simulink model "NewKitchen_REB_workstation"  (R2020b)
settings: Solver=FixedStepAuto  StartTime=sim_start  StopTime=sim_end  FixedStep=sim_interval  RelTol=1e-3
undefined symbols (not defined in the file): AmbientTem, Power1, Power2, Power3, Velocity1, Velocity2
libraries: dspswit3 x6
(part 1 of 3)
settings Model: Creator=u2159176  LastModifiedBy=u2159176
settings DebuggingCC: UnconnectedInputMsg=none  UnconnectedOutputMsg=none  UnconnectedLineMsg=none  SFMachineParentedDataDiag=error
settings ModelReferenceCC: EnableRefExpFcnMdlSchedulingChecks=off

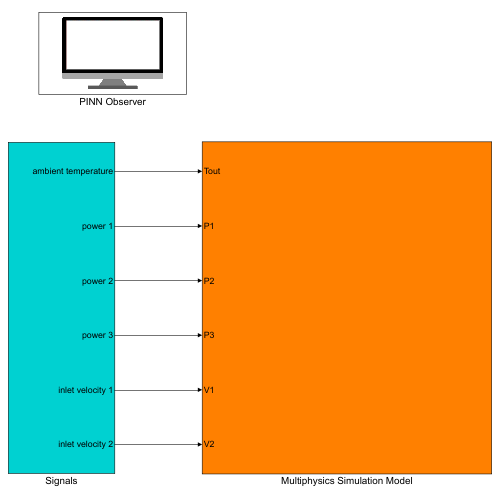
[thumbnail: Simulink's stored preview of the top-level diagram]
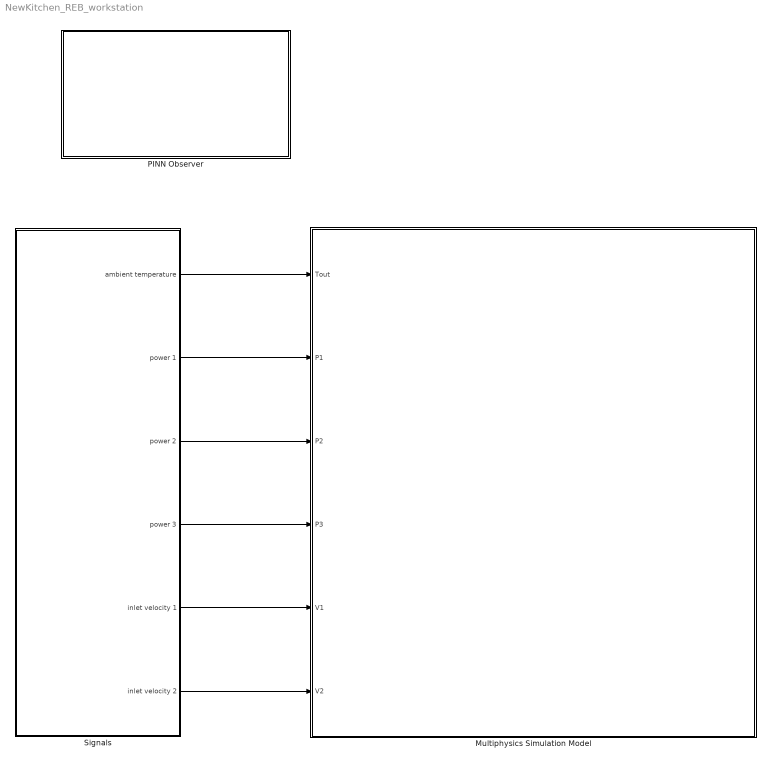
== system NewKitchen_REB_workstation ==
  Multiphysics Simulation Model : Subsystem
  PINN Observer : Subsystem
      mask Display: image('\\brio.ads.warwick.ac.uk\User68\u\u2159176\Desktop\comsol data\ECOS2023\tanshen\lcd_display.png'); % Use "Edit Image" on toolstrip to change.
  Signals : Subsystem
  wires:
  Signals/1(ambient temperature) -> Multiphysics Simulation Model/1(Tout)
  Signals/2(power 1) -> Multiphysics Simulation Model/2(P1)
  Signals/3(power 2) -> Multiphysics Simulation Model/3(P2)
  Signals/4(power 3) -> Multiphysics Simulation Model/4(P3)
  Signals/5(inlet velocity 1) -> Multiphysics Simulation Model/5(V1)
  Signals/6(inlet velocity 2) -> Multiphysics Simulation Model/6(V2)

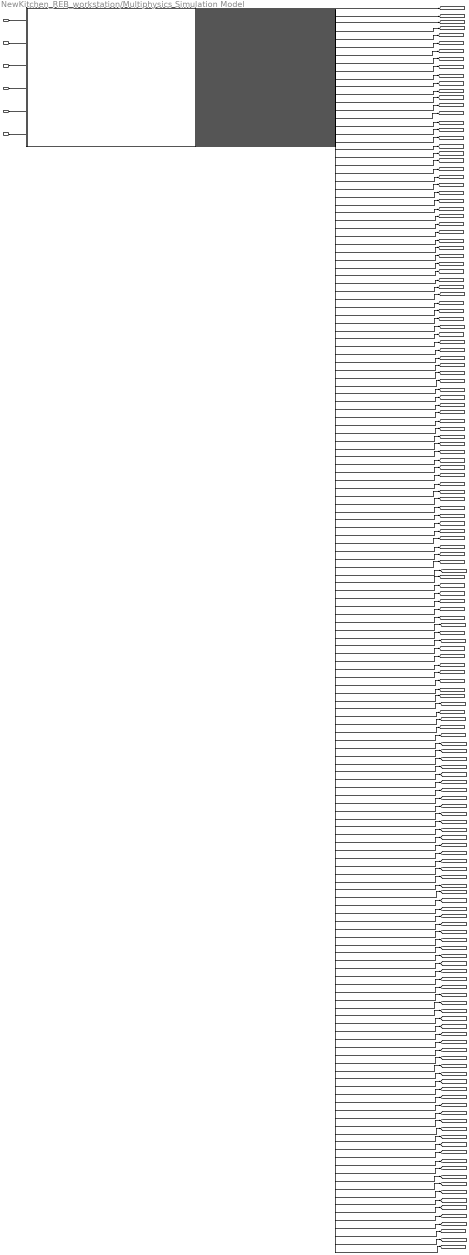
== system NewKitchen_REB_workstation/Multiphysics Simulation Model ==
  Tout : Inport
  P1 : Inport  Port=2
  P2 : Inport  Port=3
  P3 : Inport  Port=4
  V1 : Inport  Port=5
  V2 : Inport  Port=6
  COMSOL Cosimulation1 : Subsystem  mask(COMSOL Multiphysics Block){filename=\\brio.ads.warwick.ac.uk\User68\u\u2159176\Desktop\comsol data\workstation\PINN.fmu, dt=-1}
      mask prompts: dt "Communication step size"
      mask help: COMSOL Multiphysics Block version 6.2
      mask init:
      | if exist('cosimblockinit')==0
      |    error('Can not initialize block. Start COMSOL with Simulink and try again')
      | else
      |     cosimblockinit
      | end
      mask DialogControl bp Prompt: Block Parameters
      mask DialogControl bp Callback: setblockparameters
      mask Display:
      | if isempty(filename)
      |     root = char(java.lang.System.getProperty('cs.root'));
      |     if ~isempty(root)
      |         filename = fullfile(root, 'ext\LiveLink\Simulink\resources\llsimulink_comsol_logo_256.bmp');
      |         if exist(filename, 'file')
      |             im = imread(filename);
      |         end
      |     end
      | end
      | if exist('im', 'var')
      |     image(im)
      | else
      |     disp('COMSOL')
      | end
      | 
      | if exist('labels', 'var')
      |     if isfield(labels, 'in')
      |         for i=1:length(labels.in)
      |             port_label('input', i, labels.in{i})
      |         end
      |     end
      | 
      |     if isfield(labels, 'out')
      |         for i=1:length(labels.out)
      |             port_label('output', i, labels.out{i})
      |         end
      |     end
      | end
  tag scope: B110=global, B111=global, B112=global, B113=global, B114=global, B11=global, B12=global, B13=global, B14=global, B15=global, B16=global, B17=global, B18=global, B19=global, B21=global, B22=global, B23=global, B24=global, B25=global, B26=global, B27=global, B28=global, B29=global, B31=global, B32=global, B33=global, B34=global, B35=global, B36=global, B37=global, B38=global, B39=global, B410=global, B411=global, B412=global, B413=global, B414=global, B41=global, B42=global, B43=global, B44=global, B45=global, B46=global, B47=global, B48=global, B49=global, S110=global, S111=global, S112=global, S11=global, S12=global, S13=global, S14=global, S15=global, S16=global, S17=global, S18=global, S19=global, S210=global, S211=global, S212=global, S21=global, S22=global, S23=global, S24=global, S25=global, S26=global, S27=global, S28=global, S29=global, S310=global, S311=global, S312=global, S31=global, S32=global, S33=global, S34=global, S35=global, S36=global, S37=global, S38=global, S39=global, S410=global, S411=global, S412=global, S41=global, S42=global, S43=global, S44=global, S45=global, S46=global, S47=global, S48=global, S49=global, S510=global, S511=global, S512=global, S51=global, S52=global, S53=global, S54=global, S55=global, S56=global, S57=global, S58=global, S59=global, S610=global, S611=global, S612=global, S61=global, S62=global, S63=global, S64=global, S65=global, S66=global, S67=global, S68=global, S69=global, S710=global, S711=global, S712=global, S71=global, S72=global, S73=global, S74=global, S75=global, S76=global, S77=global, S78=global, S79=global, S810=global, S811=global, S812=global, S81=global, S82=global, S83=global, S84=global, S85=global, S86=global, S87=global, S88=global, S89=global, S910=global, S911=global, S912=global, S91=global, S92=global, S93=global, S94=global, S95=global, S96=global, S97=global, S98=global, S99=global, StorageTem=global, ceiling=global, dooropowall=global, neardoor=global, nearheater=global
  wires:
  COMSOL Cosimulation1/105(out105) -> [S56]
  COMSOL Cosimulation1/143(out143) -> [S88]
  COMSOL Cosimulation1/151(out151) -> [S94]
  COMSOL Cosimulation1/159(out159) -> [S912]
  COMSOL Cosimulation1/154(out154) -> [S97]
  COMSOL Cosimulation1/99(out99) -> [S412]
  COMSOL Cosimulation1/155(out155) -> [S98]
  COMSOL Cosimulation1/107(out107) -> [S58]
  COMSOL Cosimulation1/147(out147) -> [S812]
  COMSOL Cosimulation1/103(out103) -> [S54]
  COMSOL Cosimulation1/102(out102) -> [S53]
  COMSOL Cosimulation1/94(out94) -> [S47]
  COMSOL Cosimulation1/145(out145) -> [S810]
  COMSOL Cosimulation1/106(out106) -> [S57]
  COMSOL Cosimulation1/98(out98) -> [S411]
  COMSOL Cosimulation1/153(out153) -> [S96]
  COMSOL Cosimulation1/61(out61) -> [S110]
  COMSOL Cosimulation1/65(out65) -> [S22]
  COMSOL Cosimulation1/62(out62) -> [S111]
  COMSOL Cosimulation1/58(out58) -> [S17]
  COMSOL Cosimulation1/149(out149) -> [S92]
  COMSOL Cosimulation1/157(out157) -> [S910]
  COMSOL Cosimulation1/100(out100) -> [S51]
  COMSOL Cosimulation1/158(out158) -> [S911]
  COMSOL Cosimulation1/150(out150) -> [S93]
  COMSOL Cosimulation1/152(out152) -> [S95]
  COMSOL Cosimulation1/122(out122) -> [S611]
  COMSOL Cosimulation1/114(out114) -> [S63]
  COMSOL Cosimulation1/138(out138) -> [S83]
  COMSOL Cosimulation1/130(out130) -> [S77]
  COMSOL Cosimulation1/43(out43) -> [B46]
  COMSOL Cosimulation1/111(out111) -> [S512]
  COMSOL Cosimulation1/127(out127) -> [S74]
  COMSOL Cosimulation1/135(out135) -> [S712]
  COMSOL Cosimulation1/119(out119) -> [S68]
  COMSOL Cosimulation1/140(out140) -> [S85]
  COMSOL Cosimulation1/148(out148) -> [S91]
  COMSOL Cosimulation1/91(out91) -> [S44]
  COMSOL Cosimulation1/123(out123) -> [S612]
  COMSOL Cosimulation1/83(out83) -> [S38]
  COMSOL Cosimulation1/139(out139) -> [S84]
  COMSOL Cosimulation1/84(out84) -> [S39]
  COMSOL Cosimulation1/125(out125) -> [S72]
  COMSOL Cosimulation1/88(out88) -> [S41]
  COMSOL Cosimulation1/133(out133) -> [S710]
  COMSOL Cosimulation1/117(out117) -> [S66]
  COMSOL Cosimulation1/20(out20) -> [B21]
  COMSOL Cosimulation1/116(out116) -> [S65]
  COMSOL Cosimulation1/132(out132) -> [S79]
  COMSOL Cosimulation1/118(out118) -> [S67]
  COMSOL Cosimulation1/110(out110) -> [S511]
  COMSOL Cosimulation1/126(out126) -> [S73]
  COMSOL Cosimulation1/134(out134) -> [S711]
  COMSOL Cosimulation1/30(out30) -> [B32]
  COMSOL Cosimulation1/64(out64) -> [S21]
  COMSOL Cosimulation1/78(out78) -> [S33]
  COMSOL Cosimulation1/113(out113) -> [S62]
  COMSOL Cosimulation1/82(out82) -> [S37]
  COMSOL Cosimulation1/121(out121) -> [S610]
  COMSOL Cosimulation1/137(out137) -> [S82]
  COMSOL Cosimulation1/129(out129) -> [S76]
  COMSOL Cosimulation1/86(out86) -> [S311]
  COMSOL Cosimulation1/112(out112) -> [S61]
  COMSOL Cosimulation1/120(out120) -> [S69]
  COMSOL Cosimulation1/128(out128) -> [S75]
  COMSOL Cosimulation1/136(out136) -> [S81]
  COMSOL Cosimulation1/22(out22) -> [B23]
  COMSOL Cosimulation1/44(out44) -> [B47]
  COMSOL Cosimulation1/56(out56) -> [S15]
  COMSOL Cosimulation1/5(out5) -> [ceiling]
  COMSOL Cosimulation1/36(out36) -> [B38]
  COMSOL Cosimulation1/104(out104) -> [S55]
  COMSOL Cosimulation1/96(out96) -> [S49]
  COMSOL Cosimulation1/109(out109) -> [S510]
  COMSOL Cosimulation1/95(out95) -> [S48]
  COMSOL Cosimulation1/93(out93) -> [S46]
  COMSOL Cosimulation1/89(out89) -> [S42]
  COMSOL Cosimulation1/68(out68) -> [S25]
  COMSOL Cosimulation1/131(out131) -> [S78]
  COMSOL Cosimulation1/79(out79) -> [S34]
  COMSOL Cosimulation1/38(out38) -> [B41]
  COMSOL Cosimulation1/80(out80) -> [S35]
  COMSOL Cosimulation1/77(out77) -> [S32]
  COMSOL Cosimulation1/32(out32) -> [B34]
  COMSOL Cosimulation1/31(out31) -> [B33]
  COMSOL Cosimulation1/146(out146) -> [S811]
  COMSOL Cosimulation1/55(out55) -> [S14]
  COMSOL Cosimulation1/26(out26) -> [B27]
  COMSOL Cosimulation1/156(out156) -> [S99]
  COMSOL Cosimulation1/28(out28) -> [B29]
  COMSOL Cosimulation1/27(out27) -> [B28]
  COMSOL Cosimulation1/85(out85) -> [S310]
  COMSOL Cosimulation1/60(out60) -> [S19]
  COMSOL Cosimulation1/50(out50) -> [B413]
  COMSOL Cosimulation1/29(out29) -> [B31]
  COMSOL Cosimulation1/25(out25) -> [B26]
  COMSOL Cosimulation1/23(out23) -> [B24]
  COMSOL Cosimulation1/21(out21) -> [B22]
  COMSOL Cosimulation1/59(out59) -> [S18]
  COMSOL Cosimulation1/16(out16) -> [B111]
  COMSOL Cosimulation1/51(out51) -> [B414]
  COMSOL Cosimulation1/12(out12) -> [B17]
  COMSOL Cosimulation1/47(out47) -> [B410]
  COMSOL Cosimulation1/71(out71) -> [S28]
  COMSOL Cosimulation1/101(out101) -> [S52]
  COMSOL Cosimulation1/53(out53) -> [S12]
  COMSOL Cosimulation1/97(out97) -> [S410]
  COMSOL Cosimulation1/63(out63) -> [S112]
  COMSOL Cosimulation1/52(out52) -> [S11]
  COMSOL Cosimulation1/49(out49) -> [B412]
  COMSOL Cosimulation1/18(out18) -> [B113]
  COMSOL Cosimulation1/10(out10) -> [B15]
  COMSOL Cosimulation1/33(out33) -> [B35]
  COMSOL Cosimulation1/90(out90) -> [S43]
  COMSOL Cosimulation1/142(out142) -> [S87]
  COMSOL Cosimulation1/9(out9) -> [B14]
  COMSOL Cosimulation1/141(out141) -> [S86]
  COMSOL Cosimulation1/74(out74) -> [S211]
  COMSOL Cosimulation1/14(out14) -> [B19]
  COMSOL Cosimulation1/34(out34) -> [B36]
  COMSOL Cosimulation1/24(out24) -> [B25]
  COMSOL Cosimulation1/40(out40) -> [B43]
  COMSOL Cosimulation1/3(out3) -> [neardoor]
  COMSOL Cosimulation1/41(out41) -> [B44]
  COMSOL Cosimulation1/6(out6) -> [B11]
  COMSOL Cosimulation1/4(out4) -> [dooropowall]
  COMSOL Cosimulation1/67(out67) -> [S24]
  COMSOL Cosimulation1/81(out81) -> [S36]
  COMSOL Cosimulation1/115(out115) -> [S64]
  COMSOL Cosimulation1/87(out87) -> [S312]
  COMSOL Cosimulation1/48(out48) -> [B411]
  COMSOL Cosimulation1/108(out108) -> [S59]
  COMSOL Cosimulation1/54(out54) -> [S13]
  COMSOL Cosimulation1/15(out15) -> [B110]
  COMSOL Cosimulation1/46(out46) -> [B49]
  COMSOL Cosimulation1/45(out45) -> [B48]
  COMSOL Cosimulation1/8(out8) -> [B13]
  COMSOL Cosimulation1/39(out39) -> [B42]
  COMSOL Cosimulation1/42(out42) -> [B45]
  COMSOL Cosimulation1/13(out13) -> [B18]
  COMSOL Cosimulation1/19(out19) -> [B114]
  COMSOL Cosimulation1/70(out70) -> [S27]
  COMSOL Cosimulation1/72(out72) -> [S29]
  COMSOL Cosimulation1/35(out35) -> [B37]
  COMSOL Cosimulation1/2(out2) -> [nearheater]
  COMSOL Cosimulation1/124(out124) -> [S71]
  COMSOL Cosimulation1/66(out66) -> [S23]
  COMSOL Cosimulation1/37(out37) -> [B39]
  COMSOL Cosimulation1/92(out92) -> [S45]
  COMSOL Cosimulation1/69(out69) -> [S26]
  COMSOL Cosimulation1/73(out73) -> [S210]
  COMSOL Cosimulation1/144(out144) -> [S89]
  COMSOL Cosimulation1/1(out1) -> [StorageTem]
  COMSOL Cosimulation1/11(out11) -> [B16]
  COMSOL Cosimulation1/7(out7) -> [B12]
  COMSOL Cosimulation1/76(out76) -> [S31]
  COMSOL Cosimulation1/75(out75) -> [S212]
  COMSOL Cosimulation1/17(out17) -> [B112]
  COMSOL Cosimulation1/57(out57) -> [S16]
  Tout/1 -> COMSOL Cosimulation1/1(in1)
  P1/1 -> COMSOL Cosimulation1/2(in2)
  P2/1 -> COMSOL Cosimulation1/3(in3)
  P3/1 -> COMSOL Cosimulation1/4(in4)
  V1/1 -> COMSOL Cosimulation1/5(in5)
  V2/1 -> COMSOL Cosimulation1/6(in6)

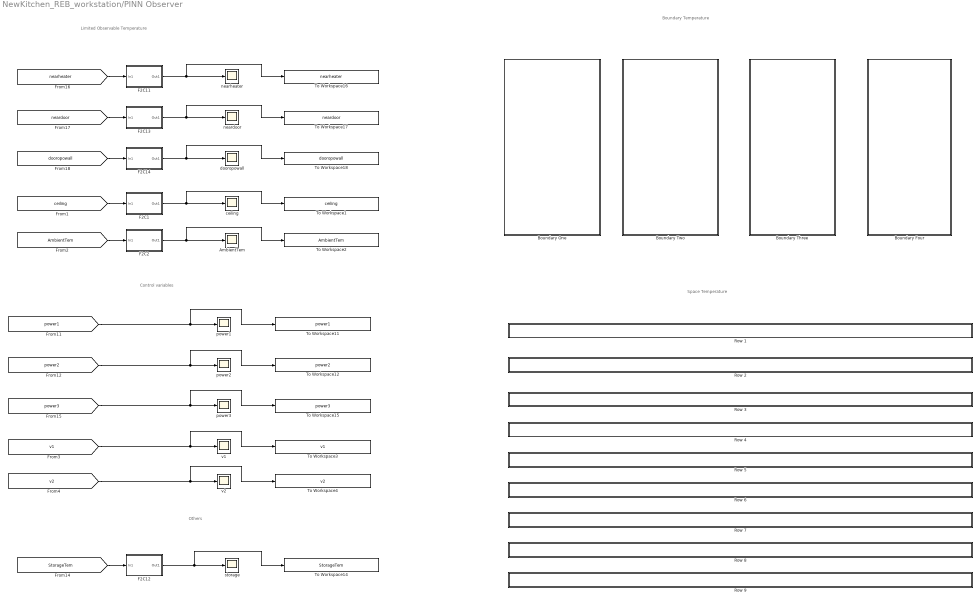
== system NewKitchen_REB_workstation/PINN Observer ==
  note: Control variables
  note: Space Temperature
  note: Limited Observable Temperature
  note: Boundary Temperature
  note: Others
  AmbientTem : Scope
  Boundary Four : Subsystem
  Boundary One : Subsystem
  Boundary Three : Subsystem
  Boundary Two : Subsystem
  F2C1 : Subsystem
  F2C11 : Subsystem
  F2C12 : Subsystem
  F2C13 : Subsystem
  F2C14 : Subsystem
  F2C2 : Subsystem
  Row 1 : Subsystem
  Row 2 : Subsystem
  Row 3 : Subsystem
  Row 4 : Subsystem
  Row 5 : Subsystem
  Row 6 : Subsystem
  Row 7 : Subsystem
  Row 8 : Subsystem
  Row 9 : Subsystem
  To Workspace1 : ToWorkspace  VariableName=ceiling  SampleTime=-1
  To Workspace11 : ToWorkspace  VariableName=power1  SampleTime=-1
  To Workspace12 : ToWorkspace  VariableName=power2  SampleTime=-1
  To Workspace14 : ToWorkspace  VariableName=StorageTem  SampleTime=-1
  To Workspace15 : ToWorkspace  VariableName=power3  SampleTime=-1
  To Workspace16 : ToWorkspace  VariableName=nearheater  SampleTime=-1
  To Workspace17 : ToWorkspace  VariableName=neardoor  SampleTime=-1
  To Workspace18 : ToWorkspace  VariableName=dooropowall  SampleTime=-1
  To Workspace2 : ToWorkspace  VariableName=AmbientTem  SampleTime=-1
  To Workspace3 : ToWorkspace  VariableName=v1  SampleTime=-1
  To Workspace4 : ToWorkspace  VariableName=v2  SampleTime=-1
  ceiling : Scope
  dooropowall : Scope
  neardoor : Scope
  nearheater : Scope
  power1 : Scope
  power2 : Scope
  power3 : Scope
  storage : Scope
  v1 : Scope
  v2 : Scope
  wires:
  [power3] -> power3/1, To Workspace15/1
  [power2] -> To Workspace12/1, power2/1
  [StorageTem] -> F2C12/1(In1)
  F2C12/1(Out1) -> To Workspace14/1, storage/1
  [power1] -> power1/1, To Workspace11/1
  [nearheater] -> F2C11/1(In1)
  F2C11/1(Out1) -> To Workspace16/1, nearheater/1
  F2C13/1(Out1) -> neardoor/1, To Workspace17/1
  [neardoor] -> F2C13/1(In1)
  [dooropowall] -> F2C14/1(In1)
  F2C14/1(Out1) -> To Workspace18/1, dooropowall/1
  F2C1/1(Out1) -> ceiling/1, To Workspace1/1
  [ceiling] -> F2C1/1(In1)
  [AmbientTem] -> F2C2/1(In1)
  F2C2/1(Out1) -> To Workspace2/1, AmbientTem/1
  [v1] -> To Workspace3/1, v1/1
  [v2] -> v2/1, To Workspace4/1

== system NewKitchen_REB_workstation/Signals ==
  AmbientTem : Subsystem
  C2F3 : Subsystem
  Power1 : Subsystem
  Power2 : Subsystem
  Power3 : Subsystem
  V1 : Subsystem
  V2 : Subsystem
  ambient temperature : Outport
  power 1 : Outport  Port=2
  power 2 : Outport  Port=3
  power 3 : Outport  Port=4
  inlet velocity 1 : Outport  Port=5
  inlet velocity 2 : Outport  Port=6
  tag scope: AmbientTem=global, power1=global, power2=global, power3=global, v1=global, v2=global
  wires:
  C2F3/1(Tout) -> ambient temperature/1, [AmbientTem]
  AmbientTem/1(signal) -> C2F3/1(signal)
  Power1/1(P1) -> power 1/1, [power1]
  V1/1(V1) -> inlet velocity 1/1, [v1]
  Power2/1(P2) -> power 2/1, [power2]
  Power3/1(P3) -> power 3/1, [power3]
  V2/1(V2) -> inlet velocity 2/1, [v2]

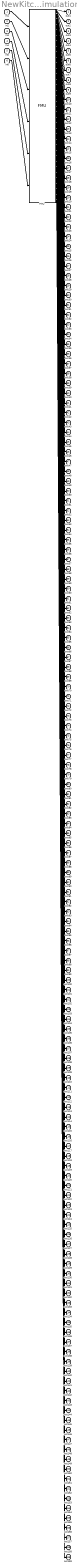
== system NewKitchen_REB_workstation/Multiphysics Simulation Model/COMSOL Cosimulation1 ==
  in1 : Inport
  in2 : Inport  Port=2
  in3 : Inport  Port=3
  in4 : Inport  Port=4
  in5 : Inport  Port=5
  in6 : Inport  Port=6
  FMU : FMU  FMUName=PINN.fmu  FMUDebugLogging=on  FMUMode=CoSimulation  Tin=292.15  mask(demo0820for62_workstation.mph [Co-Simulation, v2.0]){}
      mask Display:
      | if (exist([Simulink.fileGenControl('get','CacheFolder') '\slprj\_fmu\1c0485e634db74c5303fdcceaec22f00\PINN\model.png'],'file'))
      |     image([Simulink.fileGenControl('get','CacheFolder') '\slprj\_fmu\1c0485e634db74c5303fdcceaec22f00\PINN\model.png']);
      | else
      |     disp('demo0820for62_workstation.mph');
      | end
      | port_label('output',1,'comp1.dom1');
      | port_label('output',2,'comp1.point1');
      | port_label('output',3,'comp1.point2');
      | port_label('output',4,'comp1.point3');
      | port_label('output',5,'comp1.point4');
      | port_label('output',6,'comp1.point5');
      | port_label('output',7,'comp1.point6');
      | port_label('output',8,'comp1.point7');
      | port_label('output',9,'comp1.point8');
      | port_label('output',10,'comp1.point9');
      | port_label('output',11,'comp1.point10');
      | port_label('output',12,'comp1.point11');
      | port_label('output',13,'comp1.point12');
      | port_label('output',14,'comp1.point13');
      | port_label('output',15,'comp1.point14');
      | port_label('output',16,'comp1.point15');
      | port_label('output',17,'comp1.point16');
      | port_label('output',18,'comp1.point17');
      | port_label('output',19,'comp1.point18');
      | port_label('output',20,'comp1.point19');
      | port_label('output',21,'comp1.point20');
      | port_label('output',22,'comp1.point21');
      | port_label('output',23,'comp1.point22');
      | port_label('output',24,'comp1.point23');
      | port_label('output',25,'comp1.point24');
      | port_label('output',26,'comp1.point25');
      | port_label('output',27,'comp1.point26');
      | port_label('output',28,'comp1.point27');
      | port_label('output',29,'comp1.point28');
      | port_label('output',30,'comp1.point29');
      | port_label('output',31,'comp1.point30');
      | port_label('output',32,'comp1.point31');
      | port_label('output',33,'comp1.point32');
      | port_label('output',34,'comp1.point33');
      | port_label('output',35,'comp1.point34');
      | port_label('output',36,'comp1.point35');
      | port_label('output',37,'comp1.point36');
      | port_label('output',38,'comp1.point37');
      | port_label('output',39,'comp1.point38');
      | port_label('output',40,'comp1.point39');
      | port_label('output',41,'comp1.point40');
      | port_label('output',42,'comp1.point41');
      | port_label('output',43,'comp1.point42');
      | port_label('output',44,'comp1.point43');
      | port_label('output',45,'comp1.point44');
      | port_label('output',46,'comp1.point45');
      | port_label('output',47,'comp1.point46');
      | port_label('output',48,'comp1.point47');
      | port_label('output',49,'comp1.point48');
      | port_label('output',50,'comp1.point49');
      | port_label('output',51,'comp1.point50');
      | port_label('output',52,'comp1.point51');
      | port_label('output',53,'comp1.point52');
      | port_label('output',54,'comp1.point53');
      | port_label('output',55,'comp1.point54');
      | port_label('output',56,'comp1.point55');
      | port_label('output',57,'comp1.point56');
      | port_label('output',58,'comp1.point57');
      | port_label('output',59,'comp1.point58');
      | port_label('output',60,'comp1.point59');
      | port_label('output',61,'comp1.point60');
      | port_label('output',62,'comp1.point61');
      | port_label('output',63,'comp1.point62');
      | port_label('output',64,'comp1.point63');
      | port_label('output',65,'comp1.point64');
      | port_label('output',66,'comp1.point65');
      | port_label('output',67,'comp1.point66');
      | port_label('output',68,'comp1.point67');
      | port_label('output',69,'comp1.point68');
      | port_label('output',70,'comp1.point69');
      | port_label('output',71,'comp1.point70');
      | port_label('output',72,'comp1.point71');
      | port_label('output',73,'comp1.point72');
      | port_label('output',74,'comp1.point73');
      | port_label('output',75,'comp1.point74');
      | port_label('output',76,'comp1.point75');
      | port_label('output',77,'comp1.point76');
      | port_label('output',78,'comp1.point77');
      | port_label('output',79,'comp1.point78');
      | port_label('output',80,'comp1.point79');
      | port_label('output',81,'comp1.point80');
      | port_label('output',82,'comp1.point81');
      | port_label('output',83,'comp1.point82');
      | port_label('output',84,'comp1.point83');
      | port_label('output',85,'comp1.point84');
      | port_label('output',86,'comp1.point85');
      | port_label('output',87,'comp1.point86');
      | port_label('output',88,'comp1.point87');
      | port_label('output',89,'comp1.point88');
      | port_label('output',90,'comp1.point89');
      | port_label('output',91,'comp1.point90');
      | port_label('output',92,'comp1.point91');
      | port_label('output',93,'comp1.point92');
      | port_label('output',94,'comp1.point93');
      | port_label('output',95,'comp1.point94');
      | port_label('output',96,'comp1.point95');
      | port_label('output',97,'comp1.point96');
      | port_label('output',98,'comp1.point97');
      | port_label('output',99,'comp1.point98');
      | port_label('output',100,'comp1.point99');
      | port_label('output',101,'comp1.point100');
      | port_label('output',102,'comp1.point101');
      | port_label('output',103,'comp1.point102');
      | port_label('output',104,'comp1.point103');
      | port_label('output',105,'comp1.point104');
      | port_label('output',106,'comp1.point105');
      | port_label('output',107,'comp1.point106');
      | port_label('output',108,'comp1.point107');
      | port_label('output',109,'comp1.point108');
      | port_label('output',110,'comp1.point109');
      | port_label('output',111,'comp1.point110');
      | port_label('output',112,'comp1.point111');
      | port_label('output',113,'comp1.point112');
      | port_label('output',114,'comp1.point113');
      | port_label('output',115,'comp1.point114');
      | port_label('output',116,'comp1.point115');
      | port_label('output',117,'comp1.point116');
      | port_label('output',118,'comp1.point117');
      | port_label('output',119,'comp1.point118');
      | port_label('output',120,'comp1.point119');
      | port_label('output',121,'comp1.point120');
      | port_label('output',122,'comp1.point121');
      | port_label('output',123,'comp1.point122');
      | port_label('output',124,'comp1.point123');
      | port_label('output',125,'comp1.point124');
      | port_label('output',126,'comp1.point125');
      | port_label('output',127,'comp1.point126');
      | port_label('output',128,'comp1.point127');
      | port_label('output',129,'comp1.point128');
      | port_label('output',130,'comp1.point129');
      | port_label('output',131,'comp1.point130');
      | port_label('output',132,'comp1.point131');
      | port_label('output',133,'comp1.point132');
      | port_label('output',134,'comp1.point133');
      | port_label('output',135,'comp1.point134');
      | port_label('output',136,'comp1.point135');
      | port_label('output',137,'comp1.point136');
      | port_label('output',138,'comp1.point137');
      | port_label('output',139,'comp1.point138');
      | port_label('output',140,'comp1.point139');
      | port_label('output',141,'comp1.point140');
      | port_label('output',142,'comp1.point141');
      | port_label('output',143,'comp1.point142');
      | port_label('output',144,'comp1.point143');
      | port_label('output',145,'comp1.point144');
      | port_label('output',146,'comp1.point145');
      | port_label('output',147,'comp1.point146');
      | port_label('output',148,'comp1.point147');
      | port_label('output',149,'comp1.point148');
      | port_label('output',150,'comp1.point149');
      | port_label('output',151,'comp1.point150');
      | port_label('output',152,'comp1.point151');
      | port_label('output',153,'comp1.point152');
      | port_label('output',154,'comp1.point153');
      | port_label('output',155,'comp1.point154');
      | port_label('output',156,'comp1.point155');
      | port_label('output',157,'comp1.point156');
      | port_label('output',158,'comp1.point157');
      | port_label('output',159,'comp1.point158');
      | port_label('input',1,'Tout');
      | port_label('input',2,'P1');
      | port_label('input',3,'P2');
      | port_label('input',4,'P3');
      | port_label('input',5,'V1');
      | port_label('input',6,'V2');
  out1 : Outport
  out2 : Outport  Port=2
  out3 : Outport  Port=3
  out4 : Outport  Port=4
  out5 : Outport  Port=5
  out6 : Outport  Port=6
  out7 : Outport  Port=7
  out8 : Outport  Port=8
  out9 : Outport  Port=9
  out10 : Outport  Port=10
  out11 : Outport  Port=11
  out12 : Outport  Port=12
  out13 : Outport  Port=13
  out14 : Outport  Port=14
  out15 : Outport  Port=15
  out16 : Outport  Port=16
  out17 : Outport  Port=17
  out18 : Outport  Port=18
  out19 : Outport  Port=19
  out20 : Outport  Port=20
  out21 : Outport  Port=21
  out22 : Outport  Port=22
  out23 : Outport  Port=23
  out24 : Outport  Port=24
  out25 : Outport  Port=25
  out26 : Outport  Port=26
  out27 : Outport  Port=27
  out28 : Outport  Port=28
  out29 : Outport  Port=29
  out30 : Outport  Port=30
  out31 : Outport  Port=31
  out32 : Outport  Port=32
  out33 : Outport  Port=33
  out34 : Outport  Port=34
  out35 : Outport  Port=35
  out36 : Outport  Port=36
  out37 : Outport  Port=37
  out38 : Outport  Port=38
  out39 : Outport  Port=39
  out40 : Outport  Port=40
  out41 : Outport  Port=41
  out42 : Outport  Port=42
  out43 : Outport  Port=43
  out44 : Outport  Port=44
  out45 : Outport  Port=45
  out46 : Outport  Port=46
  out47 : Outport  Port=47
  out48 : Outport  Port=48
  out49 : Outport  Port=49
  out50 : Outport  Port=50
  out51 : Outport  Port=51
  out52 : Outport  Port=52
  out53 : Outport  Port=53
  out54 : Outport  Port=54
  out55 : Outport  Port=55
  out56 : Outport  Port=56
  out57 : Outport  Port=57
  out58 : Outport  Port=58
  out59 : Outport  Port=59
  out60 : Outport  Port=60
  out61 : Outport  Port=61
  out62 : Outport  Port=62
  out63 : Outport  Port=63
  out64 : Outport  Port=64
  out65 : Outport  Port=65
  out66 : Outport  Port=66
  out67 : Outport  Port=67
  out68 : Outport  Port=68
  out69 : Outport  Port=69
  out70 : Outport  Port=70
  out71 : Outport  Port=71
  out72 : Outport  Port=72
  out73 : Outport  Port=73
  out74 : Outport  Port=74
  out75 : Outport  Port=75
  out76 : Outport  Port=76
  out77 : Outport  Port=77
  out78 : Outport  Port=78
  out79 : Outport  Port=79
  out80 : Outport  Port=80
  out81 : Outport  Port=81
  out82 : Outport  Port=82
  out83 : Outport  Port=83
  out84 : Outport  Port=84
  out85 : Outport  Port=85
  out86 : Outport  Port=86
  out87 : Outport  Port=87
  out88 : Outport  Port=88
  out89 : Outport  Port=89
  out90 : Outport  Port=90
  out91 : Outport  Port=91
  out92 : Outport  Port=92
  out93 : Outport  Port=93
  out94 : Outport  Port=94
  out95 : Outport  Port=95
  out96 : Outport  Port=96
  out97 : Outport  Port=97
  out98 : Outport  Port=98
  out99 : Outport  Port=99
  out100 : Outport  Port=100
  out101 : Outport  Port=101
  out102 : Outport  Port=102
  out103 : Outport  Port=103
  out104 : Outport  Port=104
  out105 : Outport  Port=105
  out106 : Outport  Port=106
  out107 : Outport  Port=107
  out108 : Outport  Port=108
  out109 : Outport  Port=109
  out110 : Outport  Port=110
  out111 : Outport  Port=111
  out112 : Outport  Port=112
  out113 : Outport  Port=113
  out114 : Outport  Port=114
  out115 : Outport  Port=115
  out116 : Outport  Port=116
  out117 : Outport  Port=117
  out118 : Outport  Port=118
  out119 : Outport  Port=119
  out120 : Outport  Port=120
  out121 : Outport  Port=121
  out122 : Outport  Port=122
  out123 : Outport  Port=123
  out124 : Outport  Port=124
  out125 : Outport  Port=125
  out126 : Outport  Port=126
  out127 : Outport  Port=127
  out128 : Outport  Port=128
  out129 : Outport  Port=129
  out130 : Outport  Port=130
  out131 : Outport  Port=131
  out132 : Outport  Port=132
  out133 : Outport  Port=133
  out134 : Outport  Port=134
  out135 : Outport  Port=135
  out136 : Outport  Port=136
  out137 : Outport  Port=137
  out138 : Outport  Port=138
  out139 : Outport  Port=139
  out140 : Outport  Port=140
  out141 : Outport  Port=141
  out142 : Outport  Port=142
  out143 : Outport  Port=143
  out144 : Outport  Port=144
  out145 : Outport  Port=145
  out146 : Outport  Port=146
  out147 : Outport  Port=147
  out148 : Outport  Port=148
  out149 : Outport  Port=149
  out150 : Outport  Port=150
  out151 : Outport  Port=151
  out152 : Outport  Port=152
  out153 : Outport  Port=153
  out154 : Outport  Port=154
  out155 : Outport  Port=155
  out156 : Outport  Port=156
  out157 : Outport  Port=157
  out158 : Outport  Port=158
  out159 : Outport  Port=159
  wires:
  FMU/1 -> out1/1
  FMU/2 -> out2/1
  FMU/3 -> out3/1
  FMU/4 -> out4/1
  FMU/5 -> out5/1
  FMU/6 -> out6/1
  FMU/7 -> out7/1
  FMU/8 -> out8/1
  FMU/9 -> out9/1
  FMU/10 -> out10/1
  FMU/11 -> out11/1
  FMU/12 -> out12/1
  FMU/13 -> out13/1
  FMU/14 -> out14/1
  FMU/15 -> out15/1
  FMU/16 -> out16/1
  FMU/17 -> out17/1
  FMU/18 -> out18/1
  FMU/19 -> out19/1
  FMU/20 -> out20/1
  FMU/21 -> out21/1
  FMU/22 -> out22/1
  FMU/23 -> out23/1
  FMU/24 -> out24/1
  FMU/25 -> out25/1
  FMU/26 -> out26/1
  FMU/27 -> out27/1
  FMU/28 -> out28/1
  FMU/29 -> out29/1
  FMU/30 -> out30/1
  FMU/31 -> out31/1
  FMU/32 -> out32/1
  FMU/33 -> out33/1
  FMU/34 -> out34/1
  FMU/35 -> out35/1
  FMU/36 -> out36/1
  FMU/37 -> out37/1
  FMU/38 -> out38/1
  FMU/39 -> out39/1
  FMU/40 -> out40/1
  FMU/41 -> out41/1
  FMU/42 -> out42/1
  FMU/43 -> out43/1
  FMU/44 -> out44/1
  FMU/45 -> out45/1
  FMU/46 -> out46/1
  FMU/47 -> out47/1
  FMU/48 -> out48/1
  FMU/49 -> out49/1
  FMU/50 -> out50/1
  FMU/51 -> out51/1
  FMU/52 -> out52/1
  FMU/53 -> out53/1
  FMU/54 -> out54/1
  FMU/55 -> out55/1
  FMU/56 -> out56/1
  FMU/57 -> out57/1
  FMU/58 -> out58/1
  FMU/59 -> out59/1
  FMU/60 -> out60/1
  FMU/61 -> out61/1
  FMU/62 -> out62/1
  FMU/63 -> out63/1
  FMU/64 -> out64/1
  FMU/65 -> out65/1
  FMU/66 -> out66/1
  FMU/67 -> out67/1
  FMU/68 -> out68/1
  FMU/69 -> out69/1
  FMU/70 -> out70/1
  FMU/71 -> out71/1
  FMU/72 -> out72/1
  FMU/73 -> out73/1
  FMU/74 -> out74/1
  FMU/75 -> out75/1
  FMU/76 -> out76/1
  FMU/77 -> out77/1
  FMU/78 -> out78/1
  FMU/79 -> out79/1
  FMU/80 -> out80/1
  FMU/81 -> out81/1
  FMU/82 -> out82/1
  FMU/83 -> out83/1
  FMU/84 -> out84/1
  FMU/85 -> out85/1
  FMU/86 -> out86/1
  FMU/87 -> out87/1
  FMU/88 -> out88/1
  FMU/89 -> out89/1
  FMU/90 -> out90/1
  FMU/91 -> out91/1
  FMU/92 -> out92/1
  FMU/93 -> out93/1
  FMU/94 -> out94/1
  FMU/95 -> out95/1
  FMU/96 -> out96/1
  FMU/97 -> out97/1
  FMU/98 -> out98/1
  FMU/99 -> out99/1
  FMU/100 -> out100/1
  FMU/101 -> out101/1
  FMU/102 -> out102/1
  FMU/103 -> out103/1
  FMU/104 -> out104/1
  FMU/105 -> out105/1
  FMU/106 -> out106/1
  FMU/107 -> out107/1
  FMU/108 -> out108/1
  FMU/109 -> out109/1
  FMU/110 -> out110/1
  FMU/111 -> out111/1
  FMU/112 -> out112/1
  FMU/113 -> out113/1
  FMU/114 -> out114/1
  FMU/115 -> out115/1
  FMU/116 -> out116/1
  FMU/117 -> out117/1
  FMU/118 -> out118/1
  FMU/119 -> out119/1
  FMU/120 -> out120/1
  FMU/121 -> out121/1
  FMU/122 -> out122/1
  FMU/123 -> out123/1
  FMU/124 -> out124/1
  FMU/125 -> out125/1
  FMU/126 -> out126/1
  FMU/127 -> out127/1
  FMU/128 -> out128/1
  FMU/129 -> out129/1
  FMU/130 -> out130/1
  FMU/131 -> out131/1
  FMU/132 -> out132/1
  FMU/133 -> out133/1
  FMU/134 -> out134/1
  FMU/135 -> out135/1
  FMU/136 -> out136/1
  FMU/137 -> out137/1
  FMU/138 -> out138/1
  FMU/139 -> out139/1
  FMU/140 -> out140/1
  FMU/141 -> out141/1
  FMU/142 -> out142/1
  FMU/143 -> out143/1
  FMU/144 -> out144/1
  FMU/145 -> out145/1
  FMU/146 -> out146/1
  FMU/147 -> out147/1
  FMU/148 -> out148/1
  FMU/149 -> out149/1
  FMU/150 -> out150/1
  FMU/151 -> out151/1
  FMU/152 -> out152/1
  FMU/153 -> out153/1
  FMU/154 -> out154/1
  FMU/155 -> out155/1
  FMU/156 -> out156/1
  FMU/157 -> out157/1
  FMU/158 -> out158/1
  FMU/159 -> out159/1
  in1/1 -> FMU/1
  in2/1 -> FMU/2
  in3/1 -> FMU/3
  in4/1 -> FMU/4
  in5/1 -> FMU/5
  in6/1 -> FMU/6

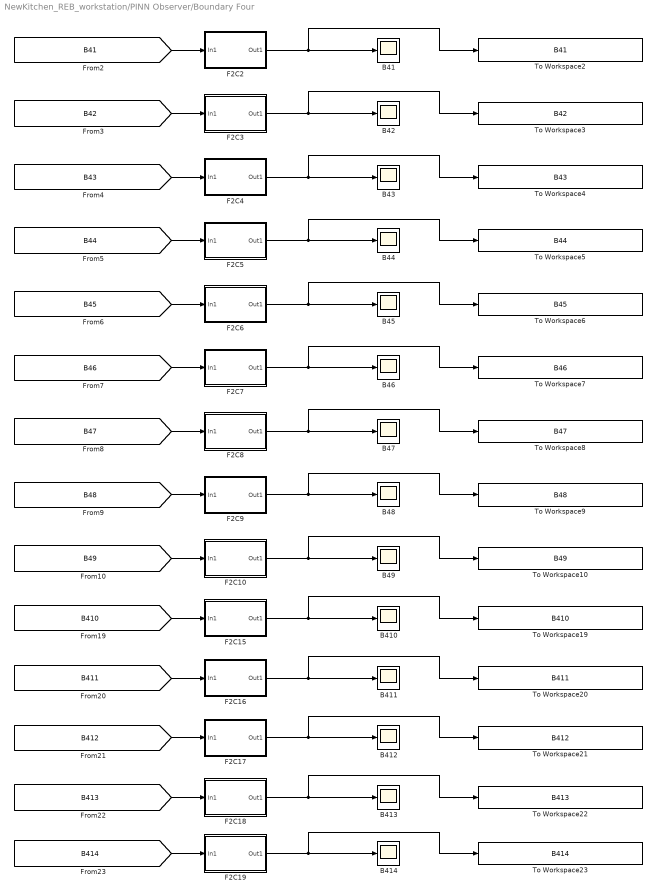
== system NewKitchen_REB_workstation/PINN Observer/Boundary Four ==
  B{41..49,410..414} (14 alike) : Scope
  F2C10 : Subsystem
  F2C15 : Subsystem
  F2C16 : Subsystem
  F2C17 : Subsystem
  F2C18 : Subsystem
  F2C19 : Subsystem
  F2C2 : Subsystem
  F2C3 : Subsystem
  F2C4 : Subsystem
  F2C5 : Subsystem
  F2C6 : Subsystem
  F2C7 : Subsystem
  F2C8 : Subsystem
  F2C9 : Subsystem
  To Workspace10 : ToWorkspace  VariableName=B49  SampleTime=-1
  To Workspace19 : ToWorkspace  VariableName=B410  SampleTime=-1
  To Workspace2 : ToWorkspace  VariableName=B41  SampleTime=-1
  To Workspace20 : ToWorkspace  VariableName=B411  SampleTime=-1
  To Workspace21 : ToWorkspace  VariableName=B412  SampleTime=-1
  To Workspace22 : ToWorkspace  VariableName=B413  SampleTime=-1
  To Workspace23 : ToWorkspace  VariableName=B414  SampleTime=-1
  To Workspace3 : ToWorkspace  VariableName=B42  SampleTime=-1
  To Workspace4 : ToWorkspace  VariableName=B43  SampleTime=-1
  To Workspace5 : ToWorkspace  VariableName=B44  SampleTime=-1
  To Workspace6 : ToWorkspace  VariableName=B45  SampleTime=-1
  To Workspace7 : ToWorkspace  VariableName=B46  SampleTime=-1
  To Workspace8 : ToWorkspace  VariableName=B47  SampleTime=-1
  To Workspace9 : ToWorkspace  VariableName=B48  SampleTime=-1
  wires:
  F2C9/1(Out1) -> B48/1, To Workspace9/1
  [B48] -> F2C9/1(In1)
  [B410] -> F2C15/1(In1)
  [B47] -> F2C8/1(In1)
  [B414] -> F2C19/1(In1)
  [B41] -> F2C2/1(In1)
  F2C17/1(Out1) -> B412/1, To Workspace21/1
  F2C10/1(Out1) -> To Workspace10/1, B49/1
  [B42] -> F2C3/1(In1)
  F2C18/1(Out1) -> To Workspace22/1, B413/1
  F2C6/1(Out1) -> To Workspace6/1, B45/1
  [B45] -> F2C6/1(In1)
  F2C16/1(Out1) -> To Workspace20/1, B411/1
  F2C8/1(Out1) -> To Workspace8/1, B47/1
  [B413] -> F2C18/1(In1)
  [B44] -> F2C5/1(In1)
  F2C19/1(Out1) -> B414/1, To Workspace23/1
  [B412] -> F2C17/1(In1)
  F2C5/1(Out1) -> B44/1, To Workspace5/1
  [B46] -> F2C7/1(In1)
  F2C15/1(Out1) -> B410/1, To Workspace19/1
  [B49] -> F2C10/1(In1)
  F2C2/1(Out1) -> To Workspace2/1, B41/1
  [B43] -> F2C4/1(In1)
  F2C3/1(Out1) -> B42/1, To Workspace3/1
  F2C7/1(Out1) -> B46/1, To Workspace7/1
  F2C4/1(Out1) -> To Workspace4/1, B43/1
  [B411] -> F2C16/1(In1)

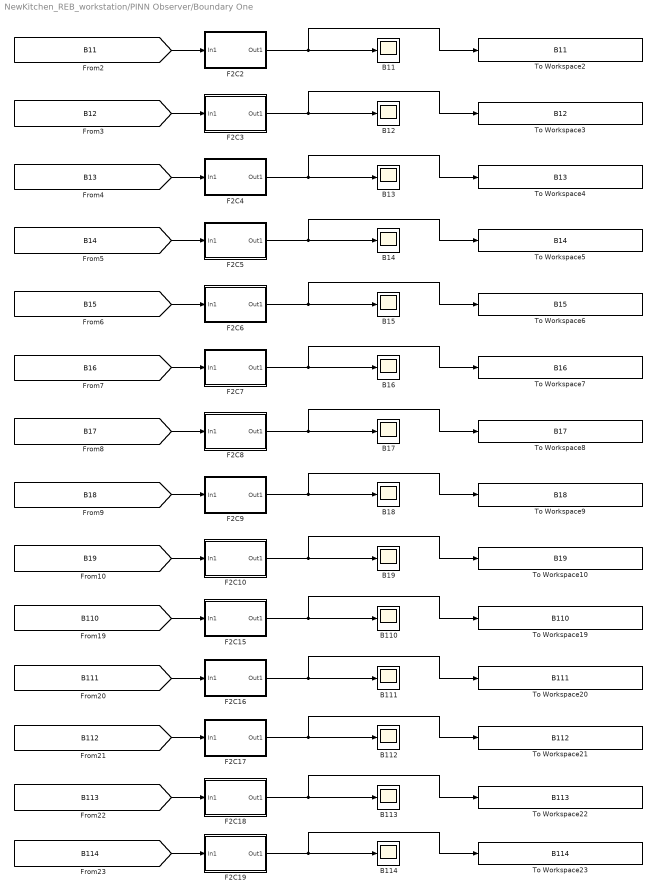
== system NewKitchen_REB_workstation/PINN Observer/Boundary One ==
  B{11..19,110..114} (14 alike) : Scope
  F2C10 : Subsystem
  F2C15 : Subsystem
  F2C16 : Subsystem
  F2C17 : Subsystem
  F2C18 : Subsystem
  F2C19 : Subsystem
  F2C2 : Subsystem
  F2C3 : Subsystem
  F2C4 : Subsystem
  F2C5 : Subsystem
  F2C6 : Subsystem
  F2C7 : Subsystem
  F2C8 : Subsystem
  F2C9 : Subsystem
  To Workspace10 : ToWorkspace  VariableName=B19  SampleTime=-1
  To Workspace19 : ToWorkspace  VariableName=B110  SampleTime=-1
  To Workspace2 : ToWorkspace  VariableName=B11  SampleTime=-1
  To Workspace20 : ToWorkspace  VariableName=B111  SampleTime=-1
  To Workspace21 : ToWorkspace  VariableName=B112  SampleTime=-1
  To Workspace22 : ToWorkspace  VariableName=B113  SampleTime=-1
  To Workspace23 : ToWorkspace  VariableName=B114  SampleTime=-1
  To Workspace3 : ToWorkspace  VariableName=B12  SampleTime=-1
  To Workspace4 : ToWorkspace  VariableName=B13  SampleTime=-1
  To Workspace5 : ToWorkspace  VariableName=B14  SampleTime=-1
  To Workspace6 : ToWorkspace  VariableName=B15  SampleTime=-1
  To Workspace7 : ToWorkspace  VariableName=B16  SampleTime=-1
  To Workspace8 : ToWorkspace  VariableName=B17  SampleTime=-1
  To Workspace9 : ToWorkspace  VariableName=B18  SampleTime=-1
  wires:
  [B111] -> F2C16/1(In1)
  F2C4/1(Out1) -> B13/1, To Workspace4/1
  F2C7/1(Out1) -> To Workspace7/1, B16/1
  F2C3/1(Out1) -> To Workspace3/1, B12/1
  [B13] -> F2C4/1(In1)
  F2C2/1(Out1) -> B11/1, To Workspace2/1
  [B19] -> F2C10/1(In1)
  F2C15/1(Out1) -> To Workspace19/1, B110/1
  [B16] -> F2C7/1(In1)
  F2C5/1(Out1) -> To Workspace5/1, B14/1
  [B112] -> F2C17/1(In1)
  F2C19/1(Out1) -> To Workspace23/1, B114/1
  [B14] -> F2C5/1(In1)
  [B113] -> F2C18/1(In1)
  F2C8/1(Out1) -> B17/1, To Workspace8/1
  F2C16/1(Out1) -> B111/1, To Workspace20/1
  [B15] -> F2C6/1(In1)
  F2C6/1(Out1) -> B15/1, To Workspace6/1
  F2C18/1(Out1) -> B113/1, To Workspace22/1
  [B12] -> F2C3/1(In1)
  F2C10/1(Out1) -> B19/1, To Workspace10/1
  F2C17/1(Out1) -> To Workspace21/1, B112/1
  [B11] -> F2C2/1(In1)
  [B114] -> F2C19/1(In1)
  [B17] -> F2C8/1(In1)
  [B110] -> F2C15/1(In1)
  [B18] -> F2C9/1(In1)
  F2C9/1(Out1) -> To Workspace9/1, B18/1

== system NewKitchen_REB_workstation/PINN Observer/Boundary Three ==
  B{31..39} (9 alike) : Scope
  F2C10 : Subsystem
  F2C2 : Subsystem
  F2C3 : Subsystem
  F2C4 : Subsystem
  F2C5 : Subsystem
  F2C6 : Subsystem
  F2C7 : Subsystem
  F2C8 : Subsystem
  F2C9 : Subsystem
  To Workspace10 : ToWorkspace  VariableName=B39  SampleTime=-1
  To Workspace2 : ToWorkspace  VariableName=B31  SampleTime=-1
  To Workspace3 : ToWorkspace  VariableName=B32  SampleTime=-1
  To Workspace4 : ToWorkspace  VariableName=B33  SampleTime=-1
  To Workspace5 : ToWorkspace  VariableName=B34  SampleTime=-1
  To Workspace6 : ToWorkspace  VariableName=B35  SampleTime=-1
  To Workspace7 : ToWorkspace  VariableName=B36  SampleTime=-1
  To Workspace8 : ToWorkspace  VariableName=B37  SampleTime=-1
  To Workspace9 : ToWorkspace  VariableName=B38  SampleTime=-1
  wires:
  F2C4/1(Out1) -> B33/1, To Workspace4/1
  F2C7/1(Out1) -> To Workspace7/1, B36/1
  F2C3/1(Out1) -> To Workspace3/1, B32/1
  [B33] -> F2C4/1(In1)
  F2C2/1(Out1) -> B31/1, To Workspace2/1
  [B39] -> F2C10/1(In1)
  [B36] -> F2C7/1(In1)
  F2C5/1(Out1) -> To Workspace5/1, B34/1
  [B34] -> F2C5/1(In1)
  F2C8/1(Out1) -> B37/1, To Workspace8/1
  [B35] -> F2C6/1(In1)
  F2C6/1(Out1) -> B35/1, To Workspace6/1
  [B32] -> F2C3/1(In1)
  F2C10/1(Out1) -> B39/1, To Workspace10/1
  [B31] -> F2C2/1(In1)
  [B37] -> F2C8/1(In1)
  [B38] -> F2C9/1(In1)
  F2C9/1(Out1) -> To Workspace9/1, B38/1

== system NewKitchen_REB_workstation/PINN Observer/Boundary Two ==
  B{21..29} (9 alike) : Scope
  F2C10 : Subsystem
  F2C2 : Subsystem
  F2C3 : Subsystem
  F2C4 : Subsystem
  F2C5 : Subsystem
  F2C6 : Subsystem
  F2C7 : Subsystem
  F2C8 : Subsystem
  F2C9 : Subsystem
  To Workspace10 : ToWorkspace  VariableName=B29  SampleTime=-1
  To Workspace2 : ToWorkspace  VariableName=B21  SampleTime=-1
  To Workspace3 : ToWorkspace  VariableName=B22  SampleTime=-1
  To Workspace4 : ToWorkspace  VariableName=B23  SampleTime=-1
  To Workspace5 : ToWorkspace  VariableName=B24  SampleTime=-1
  To Workspace6 : ToWorkspace  VariableName=B25  SampleTime=-1
  To Workspace7 : ToWorkspace  VariableName=B26  SampleTime=-1
  To Workspace8 : ToWorkspace  VariableName=B27  SampleTime=-1
  To Workspace9 : ToWorkspace  VariableName=B28  SampleTime=-1
  wires:
  F2C9/1(Out1) -> B28/1, To Workspace9/1
  [B28] -> F2C9/1(In1)
  [B27] -> F2C8/1(In1)
  [B21] -> F2C2/1(In1)
  F2C10/1(Out1) -> To Workspace10/1, B29/1
  [B22] -> F2C3/1(In1)
  F2C6/1(Out1) -> To Workspace6/1, B25/1
  [B25] -> F2C6/1(In1)
  F2C8/1(Out1) -> To Workspace8/1, B27/1
  [B24] -> F2C5/1(In1)
  F2C5/1(Out1) -> B24/1, To Workspace5/1
  [B26] -> F2C7/1(In1)
  [B29] -> F2C10/1(In1)
  F2C2/1(Out1) -> To Workspace2/1, B21/1
  [B23] -> F2C4/1(In1)
  F2C3/1(Out1) -> B22/1, To Workspace3/1
  F2C7/1(Out1) -> B26/1, To Workspace7/1
  F2C4/1(Out1) -> To Workspace4/1, B23/1

== system NewKitchen_REB_workstation/PINN Observer/F2C1 ==
  In1 : Inport
  Constant : Constant  Value=273.15
  Subtract : Sum  Inputs=+-
  Out1 : Outport
  wires:
  Subtract/1 -> Out1/1
  Constant/1 -> Subtract/2
  In1/1 -> Subtract/1

== system NewKitchen_REB_workstation/PINN Observer/F2C11 ==
  In1 : Inport
  Constant : Constant  Value=273.15
  Subtract : Sum  Inputs=+-
  Out1 : Outport
  wires:
  In1/1 -> Subtract/1
  Constant/1 -> Subtract/2
  Subtract/1 -> Out1/1

== system NewKitchen_REB_workstation/PINN Observer/F2C12 ==
  In1 : Inport
  Constant : Constant  Value=273.15
  Subtract : Sum  Inputs=+-
  Out1 : Outport
  wires:
  Subtract/1 -> Out1/1
  Constant/1 -> Subtract/2
  In1/1 -> Subtract/1

== system NewKitchen_REB_workstation/PINN Observer/F2C13 ==
  In1 : Inport
  Constant : Constant  Value=273.15
  Subtract : Sum  Inputs=+-
  Out1 : Outport
  wires:
  Subtract/1 -> Out1/1
  Constant/1 -> Subtract/2
  In1/1 -> Subtract/1

== system NewKitchen_REB_workstation/PINN Observer/F2C14 ==
  In1 : Inport
  Constant : Constant  Value=273.15
  Subtract : Sum  Inputs=+-
  Out1 : Outport
  wires:
  In1/1 -> Subtract/1
  Constant/1 -> Subtract/2
  Subtract/1 -> Out1/1

== system NewKitchen_REB_workstation/PINN Observer/F2C2 ==
  In1 : Inport
  Constant : Constant  Value=273.15
  Subtract : Sum  Inputs=+-
  Out1 : Outport
  wires:
  In1/1 -> Subtract/1
  Constant/1 -> Subtract/2
  Subtract/1 -> Out1/1

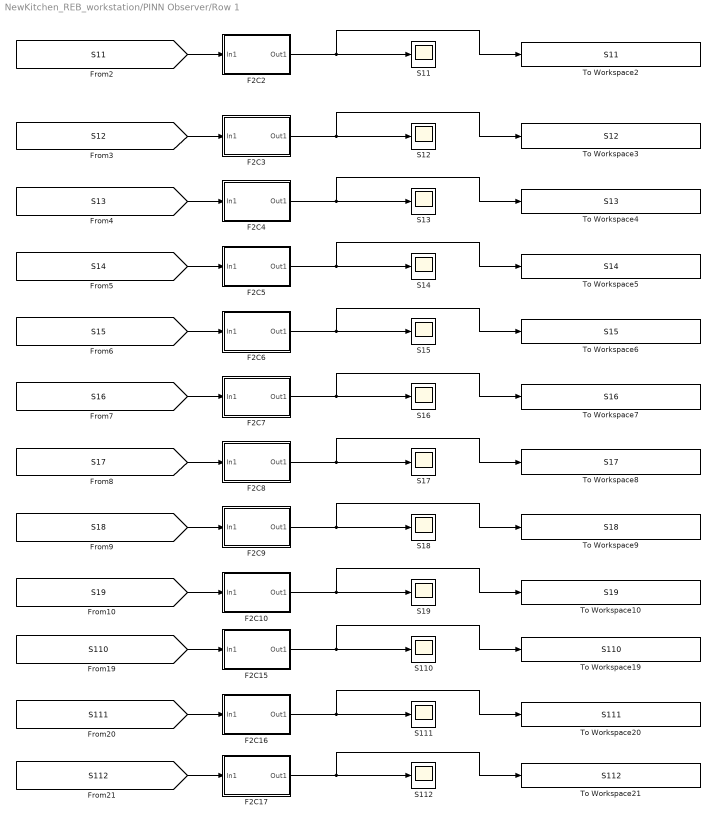
== system NewKitchen_REB_workstation/PINN Observer/Row 1 ==
  F2C10 : Subsystem
  F2C15 : Subsystem
  F2C16 : Subsystem
  F2C17 : Subsystem
  F2C2 : Subsystem
  F2C3 : Subsystem
  F2C4 : Subsystem
  F2C5 : Subsystem
  F2C6 : Subsystem
  F2C7 : Subsystem
  F2C8 : Subsystem
  F2C9 : Subsystem
  S{11..19,110..112} (12 alike) : Scope
  To Workspace10 : ToWorkspace  VariableName=S19  SampleTime=-1
  To Workspace19 : ToWorkspace  VariableName=S110  SampleTime=-1
  To Workspace2 : ToWorkspace  VariableName=S11  SampleTime=-1
  To Workspace20 : ToWorkspace  VariableName=S111  SampleTime=-1
  To Workspace21 : ToWorkspace  VariableName=S112  SampleTime=-1
  To Workspace3 : ToWorkspace  VariableName=S12  SampleTime=-1
  To Workspace4 : ToWorkspace  VariableName=S13  SampleTime=-1
  To Workspace5 : ToWorkspace  VariableName=S14  SampleTime=-1
  To Workspace6 : ToWorkspace  VariableName=S15  SampleTime=-1
  To Workspace7 : ToWorkspace  VariableName=S16  SampleTime=-1
  To Workspace8 : ToWorkspace  VariableName=S17  SampleTime=-1
  To Workspace9 : ToWorkspace  VariableName=S18  SampleTime=-1
  wires:
  [S17] -> F2C8/1(In1)
  [S19] -> F2C10/1(In1)
  F2C7/1(Out1) -> To Workspace7/1, S16/1
  F2C17/1(Out1) -> To Workspace21/1, S112/1
  [S15] -> F2C6/1(In1)
  [S112] -> F2C17/1(In1)
  F2C4/1(Out1) -> S13/1, To Workspace4/1
  F2C5/1(Out1) -> To Workspace5/1, S14/1
  [S16] -> F2C7/1(In1)
  F2C9/1(Out1) -> To Workspace9/1, S18/1
  [S110] -> F2C15/1(In1)
  F2C6/1(Out1) -> S15/1, To Workspace6/1
  F2C16/1(Out1) -> S111/1, To Workspace20/1
  F2C10/1(Out1) -> S19/1, To Workspace10/1
  [S111] -> F2C16/1(In1)
  [S18] -> F2C9/1(In1)
  F2C15/1(Out1) -> To Workspace19/1, S110/1
  [S11] -> F2C2/1(In1)
  F2C2/1(Out1) -> S11/1, To Workspace2/1
  F2C3/1(Out1) -> To Workspace3/1, S12/1
  F2C8/1(Out1) -> S17/1, To Workspace8/1
  [S13] -> F2C4/1(In1)
  [S12] -> F2C3/1(In1)
  [S14] -> F2C5/1(In1)

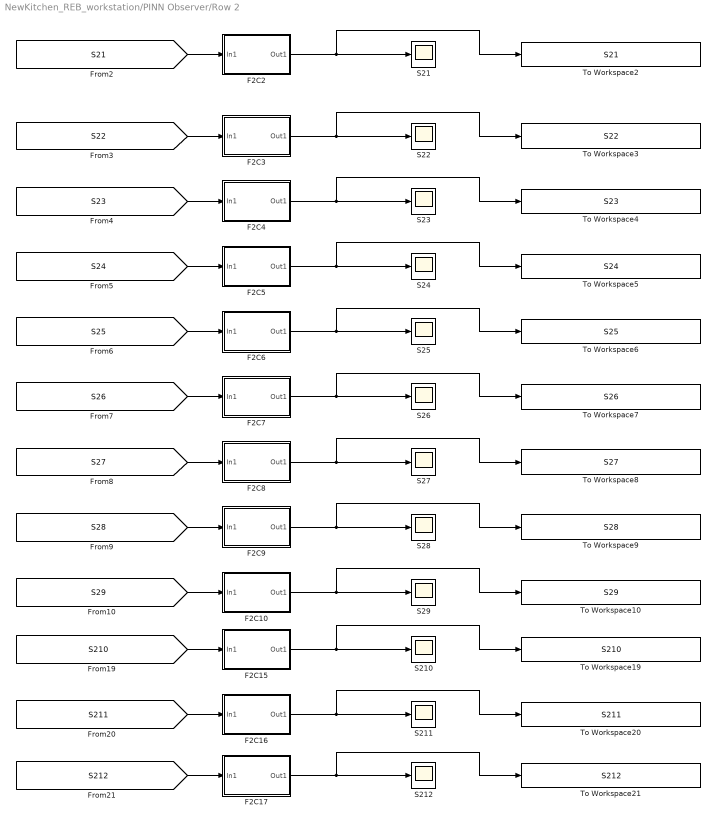
== system NewKitchen_REB_workstation/PINN Observer/Row 2 ==
  F2C10 : Subsystem
  F2C15 : Subsystem
  F2C16 : Subsystem
  F2C17 : Subsystem
  F2C2 : Subsystem
  F2C3 : Subsystem
  F2C4 : Subsystem
  F2C5 : Subsystem
  F2C6 : Subsystem
  F2C7 : Subsystem
  F2C8 : Subsystem
  F2C9 : Subsystem
  S{21..29,210..212} (12 alike) : Scope
  To Workspace10 : ToWorkspace  VariableName=S29  SampleTime=-1
  To Workspace19 : ToWorkspace  VariableName=S210  SampleTime=-1
  To Workspace2 : ToWorkspace  VariableName=S21  SampleTime=-1
  To Workspace20 : ToWorkspace  VariableName=S211  SampleTime=-1
  To Workspace21 : ToWorkspace  VariableName=S212  SampleTime=-1
  To Workspace3 : ToWorkspace  VariableName=S22  SampleTime=-1
  To Workspace4 : ToWorkspace  VariableName=S23  SampleTime=-1
  To Workspace5 : ToWorkspace  VariableName=S24  SampleTime=-1
  To Workspace6 : ToWorkspace  VariableName=S25  SampleTime=-1
  To Workspace7 : ToWorkspace  VariableName=S26  SampleTime=-1
  To Workspace8 : ToWorkspace  VariableName=S27  SampleTime=-1
  To Workspace9 : ToWorkspace  VariableName=S28  SampleTime=-1
  wires:
  [S24] -> F2C5/1(In1)
  [S22] -> F2C3/1(In1)
  [S23] -> F2C4/1(In1)
  F2C8/1(Out1) -> To Workspace8/1, S27/1
  F2C3/1(Out1) -> S22/1, To Workspace3/1
  F2C2/1(Out1) -> To Workspace2/1, S21/1
  [S21] -> F2C2/1(In1)
  F2C15/1(Out1) -> S210/1, To Workspace19/1
  [S28] -> F2C9/1(In1)
  [S211] -> F2C16/1(In1)
  F2C10/1(Out1) -> To Workspace10/1, S29/1
  F2C16/1(Out1) -> To Workspace20/1, S211/1
  F2C6/1(Out1) -> To Workspace6/1, S25/1
  [S210] -> F2C15/1(In1)
  F2C9/1(Out1) -> S28/1, To Workspace9/1
  [S26] -> F2C7/1(In1)
  F2C5/1(Out1) -> S24/1, To Workspace5/1
  F2C4/1(Out1) -> To Workspace4/1, S23/1
  [S212] -> F2C17/1(In1)
  [S25] -> F2C6/1(In1)
  F2C17/1(Out1) -> S212/1, To Workspace21/1
  F2C7/1(Out1) -> S26/1, To Workspace7/1
  [S29] -> F2C10/1(In1)
  [S27] -> F2C8/1(In1)

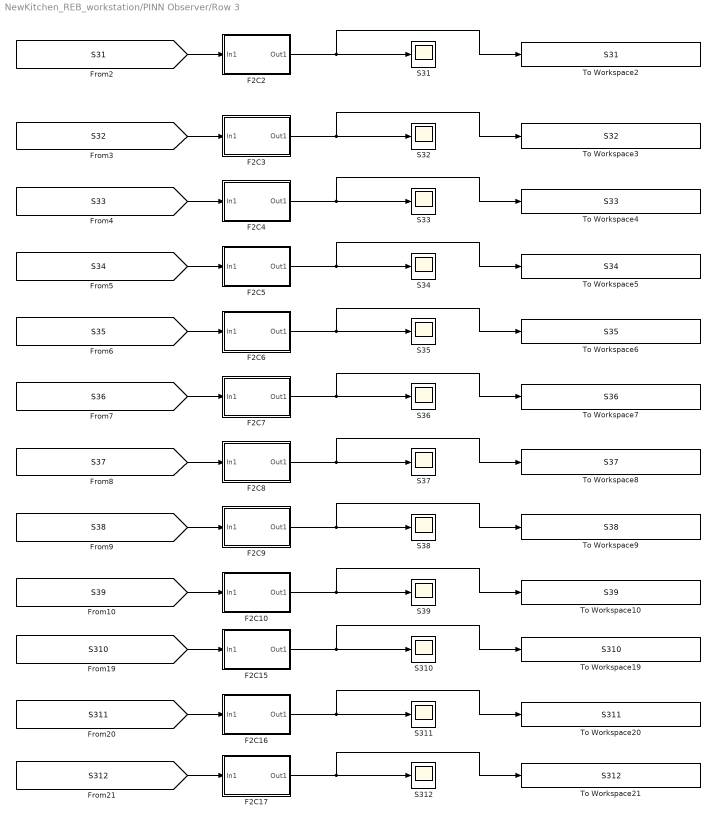
== system NewKitchen_REB_workstation/PINN Observer/Row 3 ==
  F2C10 : Subsystem
  F2C15 : Subsystem
  F2C16 : Subsystem
  F2C17 : Subsystem
  F2C2 : Subsystem
  F2C3 : Subsystem
  F2C4 : Subsystem
  F2C5 : Subsystem
  F2C6 : Subsystem
  F2C7 : Subsystem
  F2C8 : Subsystem
  F2C9 : Subsystem
  S{31..39,310..312} (12 alike) : Scope
  To Workspace10 : ToWorkspace  VariableName=S39  SampleTime=-1
  To Workspace19 : ToWorkspace  VariableName=S310  SampleTime=-1
  To Workspace2 : ToWorkspace  VariableName=S31  SampleTime=-1
  To Workspace20 : ToWorkspace  VariableName=S311  SampleTime=-1
  To Workspace21 : ToWorkspace  VariableName=S312  SampleTime=-1
  To Workspace3 : ToWorkspace  VariableName=S32  SampleTime=-1
  To Workspace4 : ToWorkspace  VariableName=S33  SampleTime=-1
  To Workspace5 : ToWorkspace  VariableName=S34  SampleTime=-1
  To Workspace6 : ToWorkspace  VariableName=S35  SampleTime=-1
  To Workspace7 : ToWorkspace  VariableName=S36  SampleTime=-1
  To Workspace8 : ToWorkspace  VariableName=S37  SampleTime=-1
  To Workspace9 : ToWorkspace  VariableName=S38  SampleTime=-1
  wires:
  [S37] -> F2C8/1(In1)
  [S39] -> F2C10/1(In1)
  F2C7/1(Out1) -> To Workspace7/1, S36/1
  F2C17/1(Out1) -> To Workspace21/1, S312/1
  [S35] -> F2C6/1(In1)
  [S312] -> F2C17/1(In1)
  F2C4/1(Out1) -> S33/1, To Workspace4/1
  F2C5/1(Out1) -> To Workspace5/1, S34/1
  [S36] -> F2C7/1(In1)
  F2C9/1(Out1) -> To Workspace9/1, S38/1
  [S310] -> F2C15/1(In1)
  F2C6/1(Out1) -> S35/1, To Workspace6/1
  F2C16/1(Out1) -> S311/1, To Workspace20/1
  F2C10/1(Out1) -> S39/1, To Workspace10/1
  [S311] -> F2C16/1(In1)
  [S38] -> F2C9/1(In1)
  F2C15/1(Out1) -> To Workspace19/1, S310/1
  [S31] -> F2C2/1(In1)
  F2C2/1(Out1) -> S31/1, To Workspace2/1
  F2C3/1(Out1) -> To Workspace3/1, S32/1
  F2C8/1(Out1) -> S37/1, To Workspace8/1
  [S33] -> F2C4/1(In1)
  [S32] -> F2C3/1(In1)
  [S34] -> F2C5/1(In1)

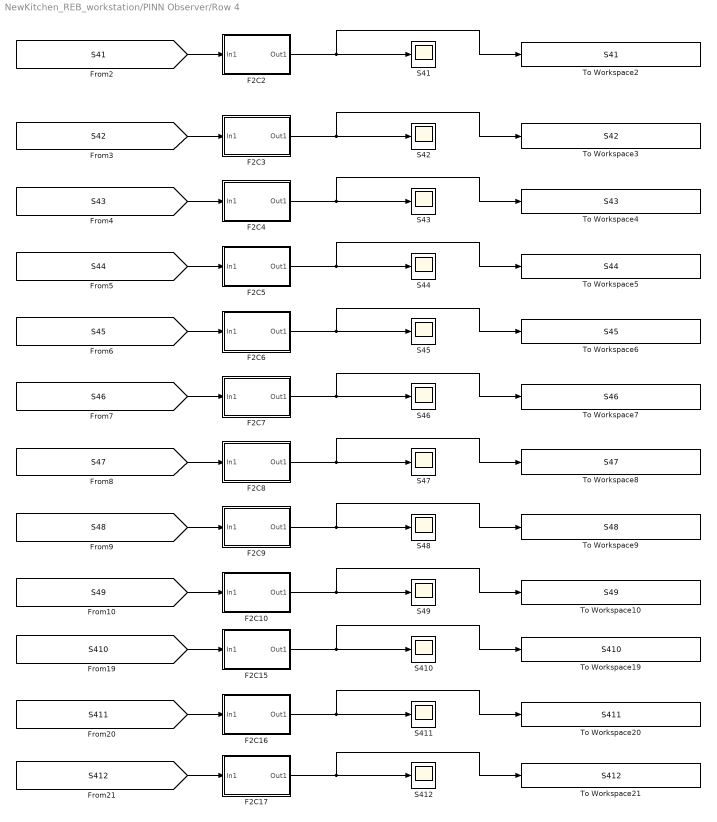
== system NewKitchen_REB_workstation/PINN Observer/Row 4 ==
  F2C10 : Subsystem
  F2C15 : Subsystem
  F2C16 : Subsystem
  F2C17 : Subsystem
  F2C2 : Subsystem
  F2C3 : Subsystem
  F2C4 : Subsystem
  F2C5 : Subsystem
  F2C6 : Subsystem
  F2C7 : Subsystem
  F2C8 : Subsystem
  F2C9 : Subsystem
  S{41..49,410..412} (12 alike) : Scope
  To Workspace10 : ToWorkspace  VariableName=S49  SampleTime=-1
  To Workspace19 : ToWorkspace  VariableName=S410  SampleTime=-1
  To Workspace2 : ToWorkspace  VariableName=S41  SampleTime=-1
  To Workspace20 : ToWorkspace  VariableName=S411  SampleTime=-1
  To Workspace21 : ToWorkspace  VariableName=S412  SampleTime=-1
  To Workspace3 : ToWorkspace  VariableName=S42  SampleTime=-1
  To Workspace4 : ToWorkspace  VariableName=S43  SampleTime=-1
  To Workspace5 : ToWorkspace  VariableName=S44  SampleTime=-1
  To Workspace6 : ToWorkspace  VariableName=S45  SampleTime=-1
  To Workspace7 : ToWorkspace  VariableName=S46  SampleTime=-1
  To Workspace8 : ToWorkspace  VariableName=S47  SampleTime=-1
  To Workspace9 : ToWorkspace  VariableName=S48  SampleTime=-1
  wires:
  [S44] -> F2C5/1(In1)
  [S42] -> F2C3/1(In1)
  [S43] -> F2C4/1(In1)
  F2C8/1(Out1) -> To Workspace8/1, S47/1
  F2C3/1(Out1) -> S42/1, To Workspace3/1
  F2C2/1(Out1) -> To Workspace2/1, S41/1
  [S41] -> F2C2/1(In1)
  F2C15/1(Out1) -> S410/1, To Workspace19/1
  [S48] -> F2C9/1(In1)
  [S411] -> F2C16/1(In1)
  F2C10/1(Out1) -> To Workspace10/1, S49/1
  F2C16/1(Out1) -> To Workspace20/1, S411/1
  F2C6/1(Out1) -> To Workspace6/1, S45/1
  [S410] -> F2C15/1(In1)
  F2C9/1(Out1) -> S48/1, To Workspace9/1
  [S46] -> F2C7/1(In1)
  F2C5/1(Out1) -> S44/1, To Workspace5/1
  F2C4/1(Out1) -> To Workspace4/1, S43/1
  [S412] -> F2C17/1(In1)
  [S45] -> F2C6/1(In1)
  F2C17/1(Out1) -> S412/1, To Workspace21/1
  F2C7/1(Out1) -> S46/1, To Workspace7/1
  [S49] -> F2C10/1(In1)
  [S47] -> F2C8/1(In1)

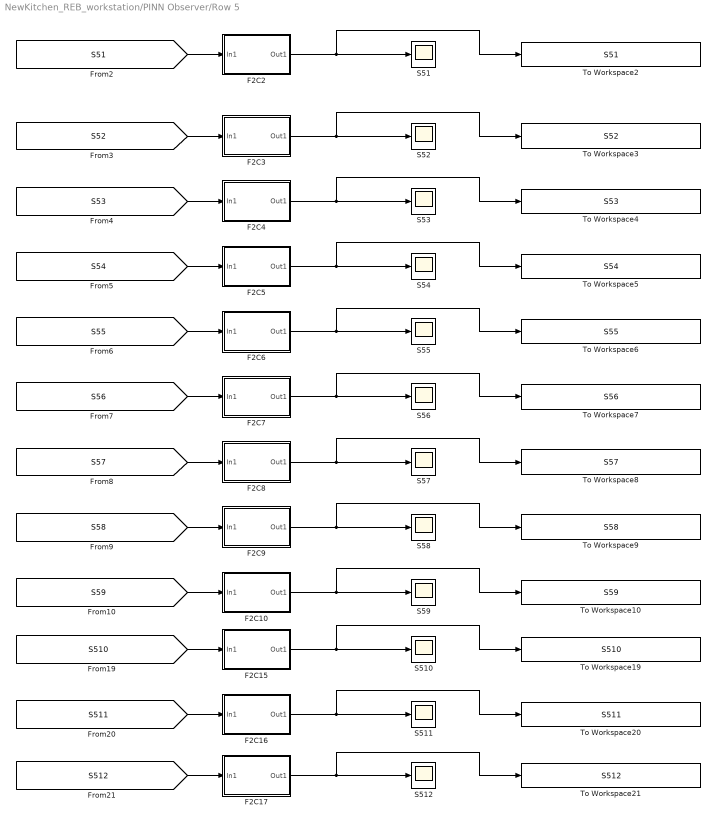
== system NewKitchen_REB_workstation/PINN Observer/Row 5 ==
  F2C10 : Subsystem
  F2C15 : Subsystem
  F2C16 : Subsystem
  F2C17 : Subsystem
  F2C2 : Subsystem
  F2C3 : Subsystem
  F2C4 : Subsystem
  F2C5 : Subsystem
  F2C6 : Subsystem
  F2C7 : Subsystem
  F2C8 : Subsystem
  F2C9 : Subsystem
  S{51..59,510..512} (12 alike) : Scope
  To Workspace10 : ToWorkspace  VariableName=S59  SampleTime=-1
  To Workspace19 : ToWorkspace  VariableName=S510  SampleTime=-1
  To Workspace2 : ToWorkspace  VariableName=S51  SampleTime=-1
  To Workspace20 : ToWorkspace  VariableName=S511  SampleTime=-1
  To Workspace21 : ToWorkspace  VariableName=S512  SampleTime=-1
  To Workspace3 : ToWorkspace  VariableName=S52  SampleTime=-1
  To Workspace4 : ToWorkspace  VariableName=S53  SampleTime=-1
  To Workspace5 : ToWorkspace  VariableName=S54  SampleTime=-1
  To Workspace6 : ToWorkspace  VariableName=S55  SampleTime=-1
  To Workspace7 : ToWorkspace  VariableName=S56  SampleTime=-1
  To Workspace8 : ToWorkspace  VariableName=S57  SampleTime=-1
  To Workspace9 : ToWorkspace  VariableName=S58  SampleTime=-1
  wires:
  [S57] -> F2C8/1(In1)
  [S59] -> F2C10/1(In1)
  F2C7/1(Out1) -> To Workspace7/1, S56/1
  F2C17/1(Out1) -> To Workspace21/1, S512/1
  [S55] -> F2C6/1(In1)
  [S512] -> F2C17/1(In1)
  F2C4/1(Out1) -> S53/1, To Workspace4/1
  F2C5/1(Out1) -> To Workspace5/1, S54/1
  [S56] -> F2C7/1(In1)
  F2C9/1(Out1) -> To Workspace9/1, S58/1
  [S510] -> F2C15/1(In1)
  F2C6/1(Out1) -> S55/1, To Workspace6/1
  F2C16/1(Out1) -> S511/1, To Workspace20/1
  F2C10/1(Out1) -> S59/1, To Workspace10/1
  [S511] -> F2C16/1(In1)
  [S58] -> F2C9/1(In1)
  F2C15/1(Out1) -> To Workspace19/1, S510/1
  [S51] -> F2C2/1(In1)
  F2C2/1(Out1) -> S51/1, To Workspace2/1
  F2C3/1(Out1) -> To Workspace3/1, S52/1
  F2C8/1(Out1) -> S57/1, To Workspace8/1
  [S53] -> F2C4/1(In1)
  [S52] -> F2C3/1(In1)
  [S54] -> F2C5/1(In1)
